simulink model "AirCtl_DesValCalc"  (R2016b)
settings: configuration reference "CodeGenConfigSet" (kept outside this file)
values from neighbouring files (symbols this model uses):
  AirCtl_ctAirTempSel_C = Calibration.Parameter    [init_AirCtl_DesValCalc.m]    (also in init_AirCtl_DesValCalc_SIL.m = Simulink.Parameter)
  AirCtl_ctEngTempSel_C = Calibration.Parameter    [init_AirCtl_DesValCalc.m]    (also in init_AirCtl_DesValCalc_SIL.m = Simulink.Parameter)
  AirCtl_facAirTempCorEOM0_MAP = Calibration.Parameter    [init_AirCtl_DesValCalc.m]    (also in init_AirCtl_DesValCalc_SIL.m = Simulink.Parameter)
  AirCtl_facAirTempCorEOM0_MAPX = Calibration.Parameter    [init_AirCtl_DesValCalc.m]    (also in init_AirCtl_DesValCalc_SIL.m = Simulink.Parameter)
  AirCtl_facAirTempCorEOM0_MAPY = Calibration.Parameter    [init_AirCtl_DesValCalc.m]    (also in init_AirCtl_DesValCalc_SIL.m = Simulink.Parameter)
  AirCtl_facEngTempCorEOM0_MAP = Calibration.Parameter    [init_AirCtl_DesValCalc.m]    (also in init_AirCtl_DesValCalc_SIL.m = Simulink.Parameter)
  AirCtl_facEngTempCorEOM0_MAPX = Calibration.Parameter    [init_AirCtl_DesValCalc.m]    (also in init_AirCtl_DesValCalc_SIL.m = Simulink.Parameter)
  AirCtl_facEngTempCorEOM0_MAPY = Calibration.Parameter    [init_AirCtl_DesValCalc.m]    (also in init_AirCtl_DesValCalc_SIL.m = Simulink.Parameter)
  AirCtl_facEnvPresCorEOM0_CUR = Calibration.Parameter    [init_AirCtl_DesValCalc.m]    (also in init_AirCtl_DesValCalc_SIL.m = Simulink.Parameter)
  AirCtl_facEnvPresCorEOM0_CURX = Calibration.Parameter    [init_AirCtl_DesValCalc.m]    (also in init_AirCtl_DesValCalc_SIL.m = Simulink.Parameter)
  AirCtl_facIndPresCorr_C = Calibration.Parameter    [init_AirCtl_DesValCalc.m]    (also in init_AirCtl_DesValCalc_SIL.m = Simulink.Parameter)
  AirCtl_mAirTempCorBasEOM0_MAP = Calibration.Parameter    [init_AirCtl_DesValCalc.m]    (also in init_AirCtl_DesValCalc_SIL.m = Simulink.Parameter)
  AirCtl_mAirTempCorBasEOM0_MAPX = Calibration.Parameter    [init_AirCtl_DesValCalc.m]    (also in init_AirCtl_DesValCalc_SIL.m = Simulink.Parameter)
  AirCtl_mAirTempCorBasEOM0_MAPY = Calibration.Parameter    [init_AirCtl_DesValCalc.m]    (also in init_AirCtl_DesValCalc_SIL.m = Simulink.Parameter)
  AirCtl_mDesBasEOM0_MAP = Calibration.Parameter    [init_AirCtl_DesValCalc.m]    (also in init_AirCtl_DesValCalc_SIL.m = Simulink.Parameter)
  AirCtl_mDesBasEOM0_MAPX = Calibration.Parameter    [init_AirCtl_DesValCalc.m]    (also in init_AirCtl_DesValCalc_SIL.m = Simulink.Parameter)
  AirCtl_mDesBasEOM0_MAPY = Calibration.Parameter    [init_AirCtl_DesValCalc.m]    (also in init_AirCtl_DesValCalc_SIL.m = Simulink.Parameter)
  AirCtl_mDesBasHiAltdEOM0_MAP = Calibration.Parameter    [init_AirCtl_DesValCalc.m]    (also in init_AirCtl_DesValCalc_SIL.m = Simulink.Parameter)
  AirCtl_mDesBasHiAltdEOM0_MAPX = Calibration.Parameter    [init_AirCtl_DesValCalc.m]    (also in init_AirCtl_DesValCalc_SIL.m = Simulink.Parameter)
  AirCtl_mDesBasHiAltdEOM0_MAPY = Calibration.Parameter    [init_AirCtl_DesValCalc.m]    (also in init_AirCtl_DesValCalc_SIL.m = Simulink.Parameter)
  AirCtl_mEngTempCorBasEOM0_MAP = Calibration.Parameter    [init_AirCtl_DesValCalc.m]    (also in init_AirCtl_DesValCalc_SIL.m = Simulink.Parameter)
  AirCtl_mEngTempCorBasEOM0_MAPX = Calibration.Parameter    [init_AirCtl_DesValCalc.m]    (also in init_AirCtl_DesValCalc_SIL.m = Simulink.Parameter)
  AirCtl_mEngTempCorBasEOM0_MAPY = Calibration.Parameter    [init_AirCtl_DesValCalc.m]    (also in init_AirCtl_DesValCalc_SIL.m = Simulink.Parameter)
  AirCtl_mMaxDesVal_C = Calibration.Parameter    [init_AirCtl_DesValCalc.m]    (also in init_AirCtl_DesValCalc_SIL.m = Simulink.Parameter)
  AirCtl_mMinDesVal_C = Calibration.Parameter    [init_AirCtl_DesValCalc.m]    (also in init_AirCtl_DesValCalc_SIL.m = Simulink.Parameter)
  AirCtl_pBstPresRef_MAP = Calibration.Parameter    [init_AirCtl_DesValCalc.m]    (also in init_AirCtl_DesValCalc_SIL.m = Simulink.Parameter)
  AirCtl_pBstPresRef_MAPX = Calibration.Parameter    [init_AirCtl_DesValCalc.m]    (also in init_AirCtl_DesValCalc_SIL.m = Simulink.Parameter)
  AirCtl_pBstPresRef_MAPY = Calibration.Parameter    [init_AirCtl_DesValCalc.m]    (also in init_AirCtl_DesValCalc_SIL.m = Simulink.Parameter)
  AirCtl_swtIndPresSel_C = Calibration.Parameter    [init_AirCtl_DesValCalc.m]    (also in init_AirCtl_DesValCalc_SIL.m = Simulink.Parameter)
settings Model: Creator=lvzhanghui  LastModifiedBy=zhulinfeng
settings ConfigSetRef: SourceLocation=Base Workspace

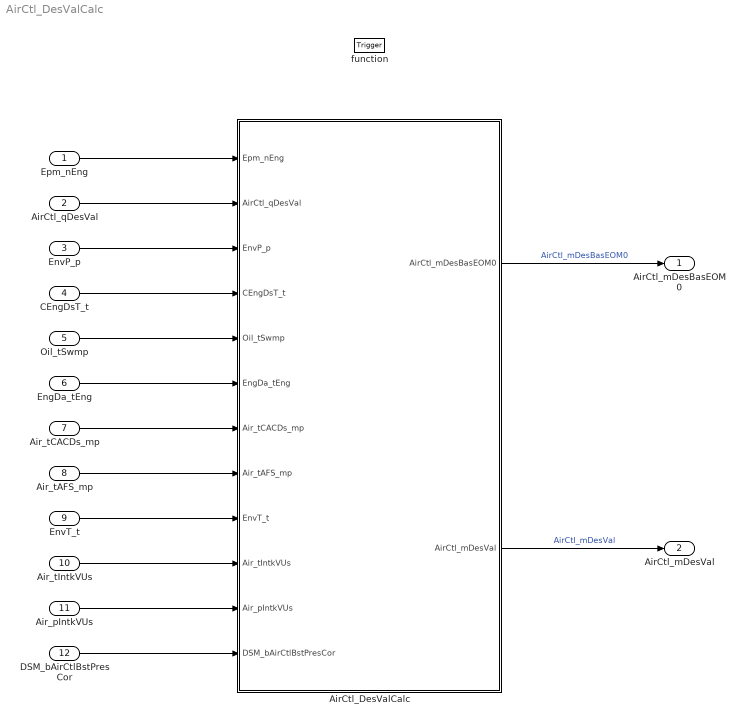
== system AirCtl_DesValCalc ==
  Epm_nEng : Inport  Tag=rpm  Description=Engine speed  OutMin=0  OutMax=6000  OutDataTypeStr=EngSpeed_rpm
  AirCtl_qDesVal : Inport  Tag=mg/hub  Description=Inner quantity for open-loop control of the exhaustgas recirculation control  Port=2  OutMin=-319  OutMax=319  OutDataTypeStr=FuelMass_mg_hub
  EnvP_p : Inport  Tag=kPa  Description=Barometric pressure  Port=3  OutMin=0  OutMax=3276  OutDataTypeStr=AirPressure_kPa
  CEngDsT_t : Inport  Tag=deg  Description=engine coolant temperature after filter  Port=4  OutMin=-200  OutMax=200  OutDataTypeStr=Temp_deg
  Oil_tSwmp : Inport  Tag=deg  Description=Oil temperature in oil sump  Port=5  OutMin=-50  OutMax=200  OutDataTypeStr=Temp_deg
  EngDa_tEng : Inport  Tag=deg  Description=Engine temperature  Port=6  OutMin=-1000  OutMax=1000  OutDataTypeStr=Temp_deg
  Air_tCACDs_mp : Inport  Tag=deg  Description=Charge-air temperature downstream from charge-air cooler  Port=7  OutMin=-200  OutMax=200  OutDataTypeStr=Temp_deg
  Air_tAFS_mp : Inport  Tag=deg  Description=Induction air temperature at the HFM  Port=8  OutMin=-200  OutMax=200  OutDataTypeStr=Temp_deg
  EnvT_t : Inport  Tag=deg  Description=Environmental temperature  Port=9  OutMin=-200  OutMax=200  OutDataTypeStr=Temp_deg
  Air_tIntkVUs : Inport  Tag=deg  Description=Intake air temperature upstream of the inlet valve  Port=10  OutMin=-200  OutMax=200  OutDataTypeStr=Temp_deg
  Air_pIntkVUs : Inport  Tag=kPa  Description=Intake valve upstream pressure  Port=11  OutMin=0  OutMax=1200  OutDataTypeStr=AirPressure_kPa
  DSM_bAirCtlBstPresCor : Inport  Description=state of Fid_AirCtlBstPresCor  Port=12  OutMin=0  OutMax=1  OutDataTypeStr=boolean
  function : TriggerPort  TriggerType=function-call  VariantControl=Variant
  AirCtl_DesValCalc : Subsystem
  AirCtl_mDesBasEOM0 : Outport  Tag=mg/hub  Description=Base air mass setpoint value from the basic map  OutMin=-15000  OutMax=15000  OutDataTypeStr=AirMass_mg_hub
  AirCtl_mDesVal : Outport  Tag=mg/hub  Description=Desired air mass  Port=2  OutMin=-15000  OutMax=15000  OutDataTypeStr=AirMass_mg_hub
  wires:
  AirCtl_DesValCalc/1(AirCtl_mDesBasEOM0) -> AirCtl_mDesBasEOM0/1  "AirCtl_mDesBasEOM0"
  AirCtl_DesValCalc/2(AirCtl_mDesVal) -> AirCtl_mDesVal/1  "AirCtl_mDesVal"
  AirCtl_qDesVal/1 -> AirCtl_DesValCalc/2(AirCtl_qDesVal)
  Epm_nEng/1 -> AirCtl_DesValCalc/1(Epm_nEng)
  EnvP_p/1 -> AirCtl_DesValCalc/3(EnvP_p)
  CEngDsT_t/1 -> AirCtl_DesValCalc/4(CEngDsT_t)
  Oil_tSwmp/1 -> AirCtl_DesValCalc/5(Oil_tSwmp)
  EngDa_tEng/1 -> AirCtl_DesValCalc/6(EngDa_tEng)
  Air_tCACDs_mp/1 -> AirCtl_DesValCalc/7(Air_tCACDs_mp)
  Air_tAFS_mp/1 -> AirCtl_DesValCalc/8(Air_tAFS_mp)
  EnvT_t/1 -> AirCtl_DesValCalc/9(EnvT_t)
  Air_tIntkVUs/1 -> AirCtl_DesValCalc/10(Air_tIntkVUs)
  Air_pIntkVUs/1 -> AirCtl_DesValCalc/11(Air_pIntkVUs)
  DSM_bAirCtlBstPresCor/1 -> AirCtl_DesValCalc/12(DSM_bAirCtlBstPresCor)

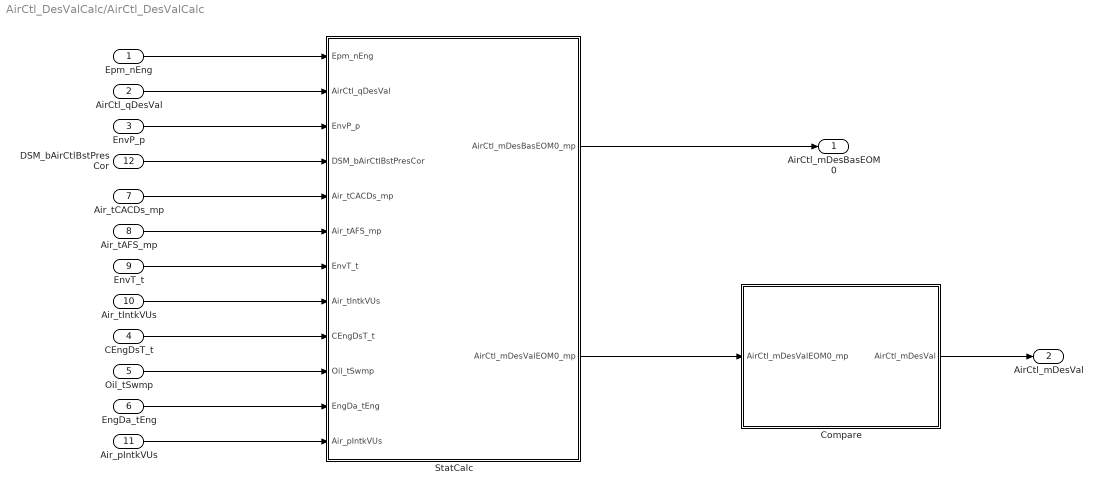
== system AirCtl_DesValCalc/AirCtl_DesValCalc ==
  Epm_nEng : Inport  Tag=rpm
  AirCtl_qDesVal : Inport  Tag=mg/hub  Port=2
  EnvP_p : Inport  Tag=kPa  Port=3
  CEngDsT_t : Inport  Tag=deg  Port=4
  Oil_tSwmp : Inport  Tag=deg  Port=5
  EngDa_tEng : Inport  Tag=deg  Port=6
  Air_tCACDs_mp : Inport  Tag=deg  Port=7
  Air_tAFS_mp : Inport  Tag=deg  Port=8
  EnvT_t : Inport  Tag=deg  Port=9
  Air_tIntkVUs : Inport  Tag=deg  Port=10
  Air_pIntkVUs : Inport  Tag=kPa  Port=11
  DSM_bAirCtlBstPresCor : Inport  Port=12
  Compare : Subsystem
  StatCalc : Subsystem
  AirCtl_mDesBasEOM0 : Outport  Tag=mg/hub
  AirCtl_mDesVal : Outport  Tag=mg/hub  Port=2
  wires:
  Epm_nEng/1 -> StatCalc/1(Epm_nEng)
  AirCtl_qDesVal/1 -> StatCalc/2(AirCtl_qDesVal)
  EnvP_p/1 -> StatCalc/3(EnvP_p)
  DSM_bAirCtlBstPresCor/1 -> StatCalc/4(DSM_bAirCtlBstPresCor)
  Air_tCACDs_mp/1 -> StatCalc/5(Air_tCACDs_mp)
  Air_tAFS_mp/1 -> StatCalc/6(Air_tAFS_mp)
  EnvT_t/1 -> StatCalc/7(EnvT_t)
  Air_tIntkVUs/1 -> StatCalc/8(Air_tIntkVUs)
  CEngDsT_t/1 -> StatCalc/9(CEngDsT_t)
  Oil_tSwmp/1 -> StatCalc/10(Oil_tSwmp)
  EngDa_tEng/1 -> StatCalc/11(EngDa_tEng)
  Air_pIntkVUs/1 -> StatCalc/12(Air_pIntkVUs)
  StatCalc/1(AirCtl_mDesBasEOM0_mp) -> AirCtl_mDesBasEOM0/1
  StatCalc/2(AirCtl_mDesValEOM0_mp) -> Compare/1(AirCtl_mDesValEOM0_mp)
  Compare/1(AirCtl_mDesVal) -> AirCtl_mDesVal/1

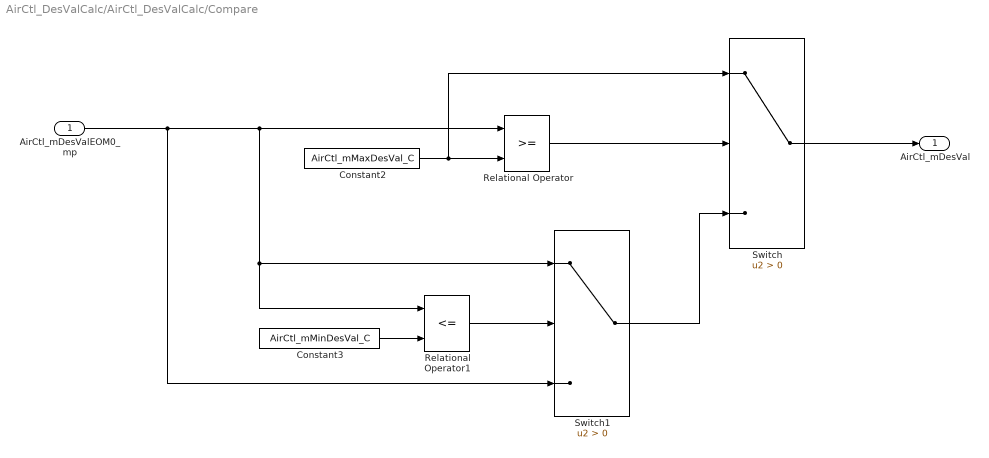
== system AirCtl_DesValCalc/AirCtl_DesValCalc/Compare ==
  AirCtl_mDesValEOM0_mp : Inport
  Constant2 : Constant  Value=AirCtl_mMaxDesVal_C
  Constant3 : Constant  Value=AirCtl_mMinDesVal_C
  Relational Operator : RelationalOperator  OutDataTypeStr=boolean  RndMeth=Simplest
  Relational Operator1 : RelationalOperator  Operator=<=  OutDataTypeStr=boolean  RndMeth=Simplest
  Switch : Switch  Criteria=u2 > Threshold
  Switch1 : Switch  Criteria=u2 > Threshold
  AirCtl_mDesVal : Outport  Tag=mg/hub
  wires:
  AirCtl_mDesValEOM0_mp/1 -> Switch1/3, Relational Operator1/1, Switch1/1, Relational Operator/1
  Relational Operator/1 -> Switch/2
  Relational Operator1/1 -> Switch1/2
  Switch1/1 -> Switch/3
  Constant2/1 -> Switch/1, Relational Operator/2
  Switch/1 -> AirCtl_mDesVal/1
  Constant3/1 -> Relational Operator1/2

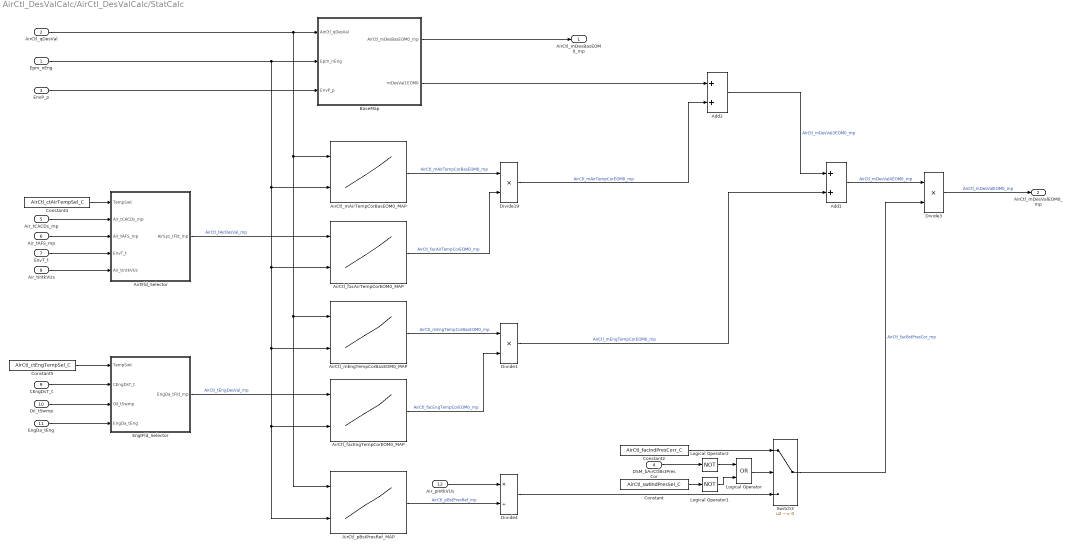
== system AirCtl_DesValCalc/AirCtl_DesValCalc/StatCalc ==
  Epm_nEng : Inport
  AirCtl_qDesVal : Inport  Port=2
  EnvP_p : Inport  Port=3
  DSM_bAirCtlBstPresCor : Inport  Port=4
  Air_tCACDs_mp : Inport  Port=5
  Air_tAFS_mp : Inport  Port=6
  EnvT_t : Inport  Port=7
  Air_tIntkVUs : Inport  Port=8
  CEngDsT_t : Inport  Port=9
  Oil_tSwmp : Inport  Port=10
  EngDa_tEng : Inport  Port=11
  Air_pIntkVUs : Inport  Port=12
  Add1 : Sum  SaturateOnIntegerOverflow=on  InputSameDT=on
  Add2 : Sum  SaturateOnIntegerOverflow=on  InputSameDT=on
  AirCtl_facAirTempCorEOM0_MAP : Lookup_n-D  BreakpointsForDimension1=AirCtl_facAirTempCorEOM0_MAPY  BreakpointsForDimension2=AirCtl_facAirTempCorEOM0_MAPX  BeginIndexSearchUsingPreviousIndexResult=on  Table=AirCtl_facAirTempCorEOM0_MAP  TableDataTypeStr=Inherit: Inherit from 'Table data'  ExtrapMethod=Clip  UseLastTableValue=on  InternalRulePriority=Speed  OutDataTypeStr=Inherit: Inherit from 'Table data'  RndMeth=Simplest  SaturateOnIntegerOverflow=on
  AirCtl_facEngTempCorEOM0_MAP : Lookup_n-D  BreakpointsForDimension1=AirCtl_facEngTempCorEOM0_MAPY  BreakpointsForDimension2=AirCtl_facEngTempCorEOM0_MAPX  BeginIndexSearchUsingPreviousIndexResult=on  Table=AirCtl_facEngTempCorEOM0_MAP  TableDataTypeStr=Inherit: Inherit from 'Table data'  ExtrapMethod=Clip  UseLastTableValue=on  InternalRulePriority=Speed  OutDataTypeStr=Inherit: Inherit from 'Table data'  RndMeth=Simplest  SaturateOnIntegerOverflow=on
  AirCtl_mAirTempCorBasEOM0_MAP : Lookup_n-D  BreakpointsForDimension1=AirCtl_mAirTempCorBasEOM0_MAPY  BreakpointsForDimension2=AirCtl_mAirTempCorBasEOM0_MAPX  BeginIndexSearchUsingPreviousIndexResult=on  Table=AirCtl_mAirTempCorBasEOM0_MAP  TableDataTypeStr=Inherit: Inherit from 'Table data'  ExtrapMethod=Clip  UseLastTableValue=on  InternalRulePriority=Speed  OutDataTypeStr=Inherit: Inherit from 'Table data'  RndMeth=Simplest  SaturateOnIntegerOverflow=on
  AirCtl_mEngTempCorBasEOM0_MAP : Lookup_n-D  BreakpointsForDimension1=AirCtl_mEngTempCorBasEOM0_MAPY  BreakpointsForDimension2=AirCtl_mEngTempCorBasEOM0_MAPX  BeginIndexSearchUsingPreviousIndexResult=on  Table=AirCtl_mEngTempCorBasEOM0_MAP  TableDataTypeStr=Inherit: Inherit from 'Table data'  ExtrapMethod=Clip  UseLastTableValue=on  InternalRulePriority=Speed  OutDataTypeStr=Inherit: Inherit from 'Table data'  RndMeth=Simplest  SaturateOnIntegerOverflow=on
  AirCtl_pBstPresRef_MAP : Lookup_n-D  BreakpointsForDimension1=AirCtl_pBstPresRef_MAPY  BreakpointsForDimension2=AirCtl_pBstPresRef_MAPX  BeginIndexSearchUsingPreviousIndexResult=on  Table=AirCtl_pBstPresRef_MAP  TableDataTypeStr=Inherit: Inherit from 'Table data'  ExtrapMethod=Clip  UseLastTableValue=on  InternalRulePriority=Speed  OutDataTypeStr=Inherit: Inherit from 'Table data'  RndMeth=Simplest  SaturateOnIntegerOverflow=on
  AirtFld_Selector : Subsystem
  BaseMap : Subsystem
  Constant : Constant  Value=AirCtl_swtIndPresSel_C
  Constant2 : Constant  Value=AirCtl_facIndPresCorr_C
  Constant4 : Constant  Value=AirCtl_ctAirTempSel_C
  Constant5 : Constant  Value=AirCtl_ctEngTempSel_C
  Divide1 : Product  Inputs=**  OutDataTypeStr=AirMass_mg_hub  SaturateOnIntegerOverflow=on
  Divide19 : Product  Inputs=**  OutDataTypeStr=Inherit: Inherit via back propagation  SaturateOnIntegerOverflow=on
  Divide3 : Product  Inputs=**  OutDataTypeStr=Inherit: Inherit via back propagation  SaturateOnIntegerOverflow=on
  Divide4 : Product  Inputs=*/  OutDataTypeStr=Factor  SaturateOnIntegerOverflow=on
  EngtFld_Selector : Subsystem
  Logical Operator : Logic  Operator=OR  AllPortsSameDT=off  OutDataTypeStr=boolean
  Logical Operator1 : Logic  Operator=NOT  AllPortsSameDT=off  OutDataTypeStr=boolean
  Logical Operator2 : Logic  Operator=NOT  AllPortsSameDT=off  OutDataTypeStr=boolean
  Switch3 : Switch  Criteria=u2 ~= 0  OutDataTypeStr=Inherit: Inherit via back propagation  SaturateOnIntegerOverflow=on  InputSameDT=on
  AirCtl_mDesBasEOM0_mp : Outport
  AirCtl_mDesValEOM0_mp : Outport  Port=2
  wires:
  Air_pIntkVUs/1 -> Divide4/1
  Divide3/1 -> AirCtl_mDesValEOM0_mp/1  "AirCtl_mDesValEOM0_mp"
  Switch3/1 -> Divide3/2  "AirCtl_facBstPresCor_mp"
  DSM_bAirCtlBstPresCor/1 -> Logical Operator2/1
  AirCtl_pBstPresRef_MAP/1 -> Divide4/2  "AirCtl_pBstPresRef_mp"
  Add1/1 -> Divide3/1  "AirCtl_mDesVal4EOM0_mp"
  Divide1/1 -> Add1/2  "AirCtl_mEngTempCorEOM0_mp"
  Divide19/1 -> Add2/2  "AirCtl_mAirTempCorEOM0_mp"
  Add2/1 -> Add1/1  "AirCtl_mDesVal3EOM0_mp"
  AirCtl_facEngTempCorEOM0_MAP/1 -> Divide1/2  "AirCtl_facEngTempCorEOM0_mp"
  AirCtl_mEngTempCorBasEOM0_MAP/1 -> Divide1/1  "AirCtl_mEngTempCorBasEOM0_mp"
  AirCtl_mAirTempCorBasEOM0_MAP/1 -> Divide19/1  "AirCtl_mAirTempCorBasEOM0_mp"
  AirCtl_facAirTempCorEOM0_MAP/1 -> Divide19/2  "AirCtl_facAirTempCorEOM0_mp"
  AirCtl_qDesVal/1 -> AirCtl_mAirTempCorBasEOM0_MAP/1, AirCtl_pBstPresRef_MAP/1, AirCtl_mEngTempCorBasEOM0_MAP/1, BaseMap/1(AirCtl_qDesVal)
  Divide4/1 -> Switch3/3
  Constant5/1 -> EngtFld_Selector/1(TempSwt)
  EngtFld_Selector/1(EngDa_tFld_mp) -> AirCtl_facEngTempCorEOM0_MAP/1  "AirCtl_tEngDesVal_mp"
  Constant4/1 -> AirtFld_Selector/1(TempSwt)
  AirtFld_Selector/1(AirSys_tFld_mp) -> AirCtl_facAirTempCorEOM0_MAP/1  "AirCtl_tAirDesVal_mp"
  Epm_nEng/1 -> AirCtl_mAirTempCorBasEOM0_MAP/2, AirCtl_facEngTempCorEOM0_MAP/2, AirCtl_pBstPresRef_MAP/2, AirCtl_mEngTempCorBasEOM0_MAP/2, AirCtl_facAirTempCorEOM0_MAP/2, BaseMap/2(Epm_nEng)
  Constant2/1 -> Switch3/1
  BaseMap/2(mDesVal1EOM0) -> Add2/1
  Logical Operator2/1 -> Logical Operator/1
  Logical Operator/1 -> Switch3/2
  Constant/1 -> Logical Operator1/1
  Logical Operator1/1 -> Logical Operator/2
  Air_tCACDs_mp/1 -> AirtFld_Selector/2(Air_tCACDs_mp)
  Air_tAFS_mp/1 -> AirtFld_Selector/3(Air_tAFS_mp)
  EnvT_t/1 -> AirtFld_Selector/4(EnvT_t)
  Air_tIntkVUs/1 -> AirtFld_Selector/5(Air_tIntkVUs)
  EnvP_p/1 -> BaseMap/3(EnvP_p)
  CEngDsT_t/1 -> EngtFld_Selector/2(CEngDsT_t)
  Oil_tSwmp/1 -> EngtFld_Selector/3(Oil_tSwmp)
  EngDa_tEng/1 -> EngtFld_Selector/4(EngDa_tEng)
  BaseMap/1(AirCtl_mDesBasEOM0_mp) -> AirCtl_mDesBasEOM0_mp/1

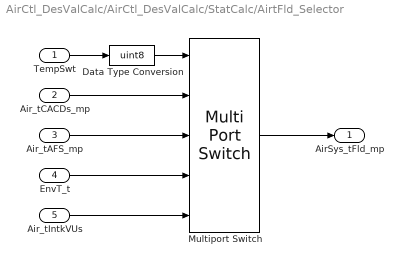
== system AirCtl_DesValCalc/AirCtl_DesValCalc/StatCalc/AirtFld_Selector ==
  TempSwt : Inport
  Air_tCACDs_mp : Inport  Tag=deg  Port=2
  Air_tAFS_mp : Inport  Tag=deg  Port=3
  EnvT_t : Inport  Tag=deg  Port=4
  Air_tIntkVUs : Inport  Tag=deg  Port=5
  Data Type Conversion : DataTypeConversion  OutDataTypeStr=uint8
  Multiport Switch : MultiPortSwitch  DataPortOrder=Zero-based contiguous  Inputs=4
  AirSys_tFld_mp : Outport  Tag=deg
  wires:
  Air_tCACDs_mp/1 -> Multiport Switch/2
  Multiport Switch/1 -> AirSys_tFld_mp/1
  EnvT_t/1 -> Multiport Switch/4
  Air_tAFS_mp/1 -> Multiport Switch/3
  Data Type Conversion/1 -> Multiport Switch/1
  TempSwt/1 -> Data Type Conversion/1
  Air_tIntkVUs/1 -> Multiport Switch/5

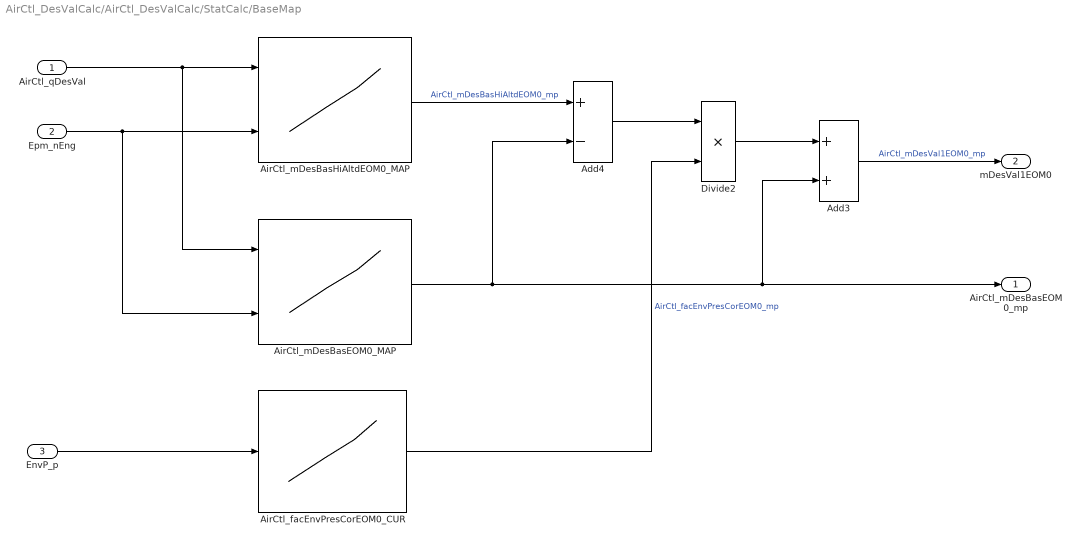
== system AirCtl_DesValCalc/AirCtl_DesValCalc/StatCalc/BaseMap ==
  AirCtl_qDesVal : Inport
  Epm_nEng : Inport  Port=2
  EnvP_p : Inport  Port=3
  Add3 : Sum  SaturateOnIntegerOverflow=on  InputSameDT=on
  Add4 : Sum  Inputs=+-  SaturateOnIntegerOverflow=on  InputSameDT=on
  AirCtl_facEnvPresCorEOM0_CUR : Lookup_n-D  NumberOfTableDimensions=1  BreakpointsForDimension1=AirCtl_facEnvPresCorEOM0_CURX  BeginIndexSearchUsingPreviousIndexResult=on  Table=AirCtl_facEnvPresCorEOM0_CUR  TableDataTypeStr=Inherit: Inherit from 'Table data'  ExtrapMethod=Clip  UseLastTableValue=on  InternalRulePriority=Speed  OutDataTypeStr=Inherit: Inherit from 'Table data'  RndMeth=Simplest  SaturateOnIntegerOverflow=on
  AirCtl_mDesBasEOM0_MAP : Lookup_n-D  BreakpointsForDimension1=AirCtl_mDesBasEOM0_MAPY  BreakpointsForDimension2=AirCtl_mDesBasEOM0_MAPX  BeginIndexSearchUsingPreviousIndexResult=on  Table=AirCtl_mDesBasEOM0_MAP  TableDataTypeStr=Inherit: Inherit from 'Table data'  ExtrapMethod=Clip  UseLastTableValue=on  InternalRulePriority=Speed  OutDataTypeStr=Inherit: Inherit from 'Table data'  RndMeth=Simplest  SaturateOnIntegerOverflow=on
  AirCtl_mDesBasHiAltdEOM0_MAP : Lookup_n-D  BreakpointsForDimension1=AirCtl_mDesBasHiAltdEOM0_MAPY  BreakpointsForDimension2=AirCtl_mDesBasHiAltdEOM0_MAPX  BeginIndexSearchUsingPreviousIndexResult=on  Table=AirCtl_mDesBasHiAltdEOM0_MAP  TableDataTypeStr=Inherit: Inherit from 'Table data'  ExtrapMethod=Clip  UseLastTableValue=on  InternalRulePriority=Speed  OutDataTypeStr=Inherit: Inherit from 'Table data'  RndMeth=Simplest  SaturateOnIntegerOverflow=on
  Divide2 : Product  Inputs=**  OutDataTypeStr=Inherit: Inherit via back propagation  SaturateOnIntegerOverflow=on
  AirCtl_mDesBasEOM0_mp : Outport
  mDesVal1EOM0 : Outport  Port=2
  wires:
  AirCtl_qDesVal/1 -> AirCtl_mDesBasHiAltdEOM0_MAP/1, AirCtl_mDesBasEOM0_MAP/1
  Epm_nEng/1 -> AirCtl_mDesBasEOM0_MAP/2, AirCtl_mDesBasHiAltdEOM0_MAP/2
  EnvP_p/1 -> AirCtl_facEnvPresCorEOM0_CUR/1
  AirCtl_mDesBasEOM0_MAP/1 -> Add4/2, Add3/2, AirCtl_mDesBasEOM0_mp/1
  Add4/1 -> Divide2/1
  Add3/1 -> mDesVal1EOM0/1  "AirCtl_mDesVal1EOM0_mp"
  AirCtl_facEnvPresCorEOM0_CUR/1 -> Divide2/2  "AirCtl_facEnvPresCorEOM0_mp"
  AirCtl_mDesBasHiAltdEOM0_MAP/1 -> Add4/1  "AirCtl_mDesBasHiAltdEOM0_mp"
  Divide2/1 -> Add3/1

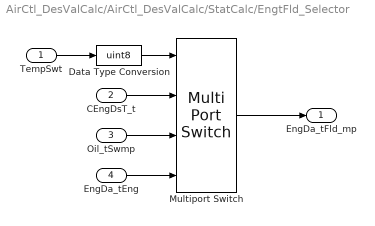
== system AirCtl_DesValCalc/AirCtl_DesValCalc/StatCalc/EngtFld_Selector ==
  TempSwt : Inport
  CEngDsT_t : Inport  Tag=deg  Port=2
  Oil_tSwmp : Inport  Tag=deg  Port=3
  EngDa_tEng : Inport  Tag=deg  Port=4
  Data Type Conversion : DataTypeConversion  OutDataTypeStr=uint8
  Multiport Switch : MultiPortSwitch  DataPortOrder=Zero-based contiguous
  EngDa_tFld_mp : Outport  Tag=deg
  wires:
  CEngDsT_t/1 -> Multiport Switch/2
  Multiport Switch/1 -> EngDa_tFld_mp/1
  EngDa_tEng/1 -> Multiport Switch/4
  Oil_tSwmp/1 -> Multiport Switch/3
  Data Type Conversion/1 -> Multiport Switch/1
  TempSwt/1 -> Data Type Conversion/1
